simulink model "modelo_NL_DH_CL_pre_restauracao_2026-06-09"  (R2025b)
settings: Solver=ode4  StartTime=0.0  StopTime=60  FixedStep=SampleTime  RelTol=1e-3
undefined symbols (not defined in the file): att_alt, C_alt, C_phi, C_theta, C_vel, h_ref, h_step_final, h_step_init, h_step_t, K_heading, Kp, Kq, Kr, phi_step_final, phi_step_init, phi_step_t, psi_ref_final, psi_ref_init, psi_ref_t, theta_ref_clamp, theta_step_final, theta_step_init, theta_step_t, TrimInput, VT_ref, Xe
libraries: slpidlib x4
settings Model: SimulationMode=accelerator  Creator=anade  LastModifiedBy=kauemartinsdesouza
settings SolverCC: ZeroCrossAlgorithm=Adaptive
settings DebuggingCC: AlgebraicLoopMsg=none  IgnoredZcDiagnostic=none

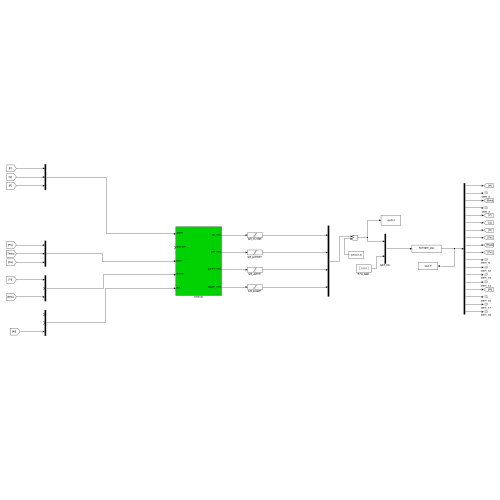
[thumbnail: Simulink's stored preview of the top-level diagram]
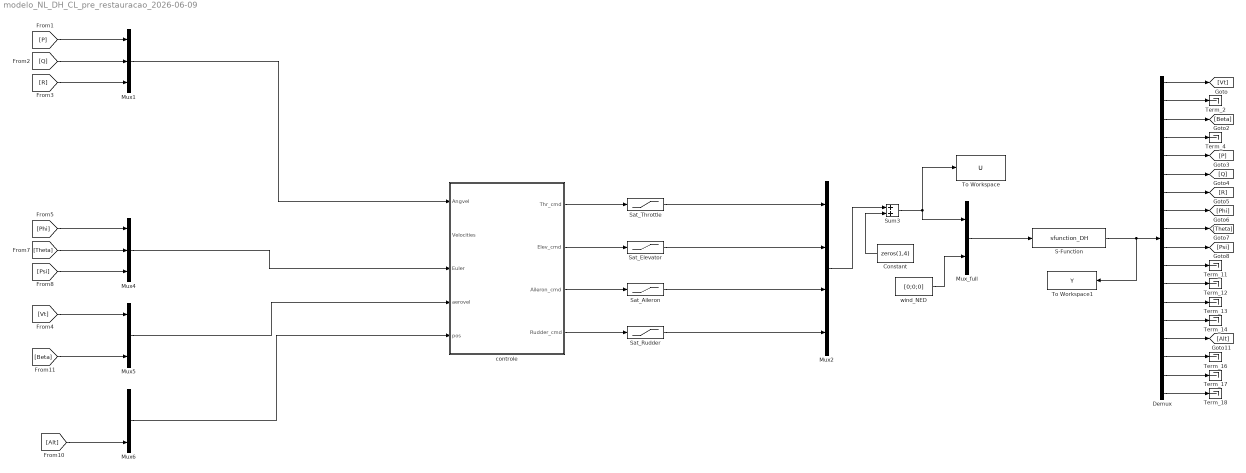
== system modelo_NL_DH_CL_pre_restauracao_2026-06-09 ==
  Constant : Constant  Value=zeros(1,4)
  Demux : Demux  Outputs=18
  Mux{1,4..6} (4 alike) : Mux  Inputs=3
  Mux2 : Mux
  Mux_full : Mux  Inputs=2
  S-Function : S-Function  FunctionName=sfunction_DH  Parameters=Xe  SFunctionDeploymentMode=off  EnableBusSupport=off
  Sat_Aileron : Saturate  UpperLimit=0.4363  LowerLimit=-0.4363
  Sat_Elevator : Saturate  UpperLimit=0.4363  LowerLimit=-0.4363
  Sat_Rudder : Saturate  UpperLimit=0.4363  LowerLimit=-0.4363
  Sat_Throttle : Saturate  UpperLimit=1  LowerLimit=0
  Sum3 : Sum
  Term_{2,4,11..14,16..18} (9 alike) : Terminator
  To Workspace : ToWorkspace  VariableName=U  SaveFormat=Structure With Time  SampleTime=-1
  To Workspace1 : ToWorkspace  VariableName=Y  SaveFormat=Structure With Time  SampleTime=-1
  controle : Subsystem
  wind_NED : Constant  Value=[0;0;0]
  wires:
  [Theta] -> Mux4/2
  Mux1/1 -> controle/1(Angvel)
  [Alt] -> Mux6/3
  [P] -> Mux1/1
  Mux4/1 -> controle/3(Euler)
  [R] -> Mux1/3
  [Phi] -> Mux4/1
  Mux6/1 -> controle/5(pos)
  [Q] -> Mux1/2
  Mux5/1 -> controle/4(aerovel)
  [Psi] -> Mux4/3
  [Beta] -> Mux5/3
  [Vt] -> Mux5/1
  controle/1(Thr_cmd) -> Sat_Throttle/1
  controle/2(Elev_cmd) -> Sat_Elevator/1
  controle/3(Aileron_cmd) -> Sat_Aileron/1
  controle/4(Rudder_cmd) -> Sat_Rudder/1
  Sat_Throttle/1 -> Mux2/1
  Sat_Elevator/1 -> Mux2/2
  Sat_Aileron/1 -> Mux2/3
  Sat_Rudder/1 -> Mux2/4
  Mux2/1 -> Sum3/1
  Constant/1 -> Sum3/2
  Sum3/1 -> Mux_full/1, To Workspace/1
  wind_NED/1 -> Mux_full/2
  Mux_full/1 -> S-Function/1
  S-Function/1 -> Demux/1, To Workspace1/1
  Demux/1 -> [Vt]
  Demux/2 -> Term_2/1
  Demux/3 -> [Beta]
  Demux/4 -> Term_4/1
  Demux/5 -> [P]
  Demux/6 -> [Q]
  Demux/7 -> [R]
  Demux/8 -> [Phi]
  Demux/9 -> [Theta]
  Demux/10 -> [Psi]
  Demux/11 -> Term_11/1
  Demux/12 -> Term_12/1
  Demux/13 -> Term_13/1
  Demux/14 -> Term_14/1
  Demux/15 -> [Alt]
  Demux/16 -> Term_16/1
  Demux/17 -> Term_17/1
  Demux/18 -> Term_18/1

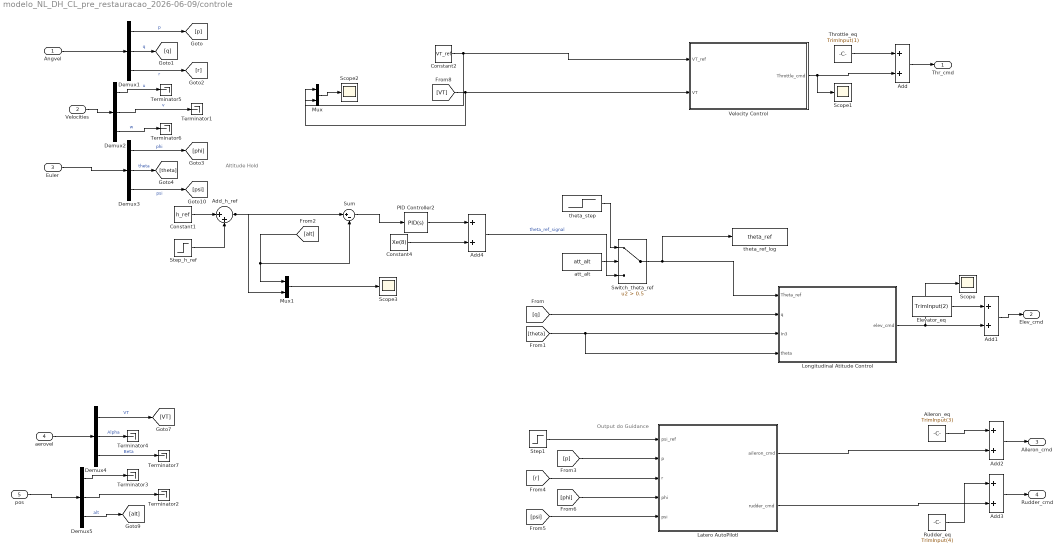
== system modelo_NL_DH_CL_pre_restauracao_2026-06-09/controle ==
  note: Altitude Hold
  note: Output do Guidance
  Angvel : Inport
  Velocities : Inport  Port=2
  Euler : Inport  Port=3
  aerovel : Inport  Port=4
  pos : Inport  Port=5
  Add{,1..4} (5 alike) : Sum
  Add_h_ref : Sum  Inputs=|++
  Aileron_eq : Constant  Value=TrimInput(3)
  Constant1 : Constant  Value=h_ref
  Constant2 : Constant  Value=VT_ref
  Constant4 : Constant  Value=Xe(8)
  Demux{1..5} (5 alike) : Demux  Outputs=3
  Elevator_eq : Constant  Value=TrimInput(2)
  Latero AutoPilotl : Subsystem
  Longitudinal Atitude Control : Subsystem
  Mux : Mux  Inputs=2
  Mux1 : Mux  Inputs=2
  PID Controller2 : slpidlib/PID Controller  Controller=PID  Form=Parallel  TimeDomain=Continuous-time  UseExternalTs=off  SampleTime=-1  IntegratorMethod=Forward Euler  FilterMethod=Forward Euler  ControllerParametersSource=internal  P=C_alt.Kp  I=C_alt.Ki  UseKiTs=off  D=C_alt.Kd  UseExternalDerivativeSource=off  N=C_alt.N  UseFilter=on  TunerSelectOption=Transfer Function Based (PID Tuner App)  InitialConditionSource=internal  InitialConditionForIntegrator=0  InitialConditionForFilter=0  DifferentiatorICPrevScaledInput=0  ExternalReset=none  TrackingMode=off  Kt=1  LimitOutput=on  SatLimitsSource=internal  UpperSaturationLimit=theta_ref_clamp(2)  LowerSaturationLimit=theta_ref_clamp(1)  LinearizeAsGain=on  AntiWindupMode=clamping  Kb=1  LimitIntegrator=off  UpperIntegratorSaturationLimit=inf  LowerIntegratorSaturationLimit=-inf  POutMin=[]  POutMax=[]  IOutMin=[]  IOutMax=[]  DOutMin=[]  DOutMax=[]  NOutMin=[]  NOutMax=[]  SumOutMin=[]  SumOutMax=[]  SaturationOutMin=[]  SaturationOutMax=[]  PParamMin=[]  PParamMax=[]  IParamMin=[]  IParamMax=[]  DParamMin=[]  DParamMax=[]  NParamMin=[]  NParamMax=[]  KbParamMin=[]  KbParamMax=[]  KtParamMin=[]  KtParamMax=[]  KbOutMin=[]  KbOutMax=[]  KtOutMin=[]  KtOutMax=[]  IntegratorOutMin=[]  IntegratorOutMax=[]  FilterOutMin=[]  FilterOutMax=[]  SumI1OutMin=[]  SumI1OutMax=[]  SumI2OutMin=[]  SumI2OutMax=[]  SumI3OutMin=[]  SumI3OutMax=[]  SumI4OutMin=[]  SumI4OutMax=[]  SumDOutMin=[]  SumDOutMax=[]  DifferentiatorOutMin=[]  DifferentiatorOutMax=[]  FilterDiffOutCoefMin=[]  FilterDiffOutCoefMax=[]  ReciprocalOutMin=[]  ReciprocalOutMax=[]  SumDenOutMin=[]  SumDenOutMax=[]  SumNumOutMin=[]  SumNumOutMax=[]  DivideOutMin=[]  DivideOutMax=[]  UdiffTsProdOutMin=[]  UdiffTsProdOutMax=[]  NTsProdOutMin=[]  NTsProdOutMax=[]  UintegralTsProdOutMin=[]  UintegralTsProdOutMax=[]  UngainTsProdOutMin=[]  UngainTsProdOutMax=[]  ClampingZeroOutDataTypeStr=Inherit: Inherit via back propagation  ClampingZeroOutMin=[]  ClampingZeroOutMax=[]  FilterDenConstantOutDataTypeStr=Inherit: Inherit via back propagation  FilterDenConstantOutMin=[]  FilterDenConstantOutMax=[]  PCopyOutDataTypeStr=Inherit: Inherit via back propagation  PCopyOutMin=[]  PCopyOutMax=[]  NCopyOutDataTypeStr=Inherit: Inherit via back propagation  NCopyOutMin=[]  NCopyOutMax=[]  IntegratorContinuousStateAttributes=''  IntegratorStateMustResolveToSignalObject=off  IntegratorRTWStateStorageClass=Auto  FilterContinuousStateAttributes=''  FilterStateMustResolveToSignalObject=off  FilterRTWStateStorageClass=Auto  ParallelPVariant=InternalParameters  IdealPVariant=Disabled  IVariant=InternalParameters  DVariant=InternalParameters  IntegratorVariant=Continuous  SatVariant=Enabled  AWVariant=ContClampingParallel  PCopyVariant=Disabled  TRVariant=Disabled  FdbkBlocksVariant=Forward  IdealPFdbkVariant=Disabled  SatFdbkVariant=Disabled  DerivativeFilterVariant=ContFilter  NVariant=InternalParameters  NCopyVariant=Disabled  FilterICVariant=InternalICsFilter  IntegratorICVariant=InternalICs  ExternalResetVariant=Disabled  TRSumVariant=Passthrough  SumFdbkVariant=Disabled  SumVariant=Sum_PID  TsampFilterVariant=InternalTs  TsampNgainVariant=Passthrough  TsampIntegralVariant=Disabled_SignalSpec  ExternalSaturationOutDataTypeStr=Inherit: Same as second input  DerivativeSourceVariant=ErrorSignal  PreIntVariant=InternalPreInt
  Rudder_eq : Constant  Value=TrimInput(4)
  Scope{,1..3} (4 alike) : Scope
      Scope settings: ActiveDisplayYMinimum=-1E-5  ActiveDisplayYMaximum=0.0001
      Scope1 settings: ActiveDisplayYMinimum=-746.9186  ActiveDisplayYMaximum=116.1605  DataLoggingVariableName=ScopeData2
      Scope2 settings: ActiveDisplayYMinimum=-70.825855594492936  ActiveDisplayYMaximum=79.160614638107518  DataLoggingVariableName=ScopeData4
      Scope3 settings: ActiveDisplayYMinimum=597.76222665286957  ActiveDisplayYMaximum=600.92459404043439  DataLoggingVariableName=ScopeData6
  Step1 : Step  Time=psi_ref_t  Before=psi_ref_init  After=psi_ref_final  SampleTime=0
  Step_h_ref : Step  Time=h_step_t  Before=h_step_init  After=h_step_final  SampleTime=0
  Sum : Sum  Inputs=|+-
  Switch_theta_ref : Switch  Criteria=u2 > Threshold  Threshold=0.5  SaturateOnIntegerOverflow=off  InputSameDT=off
  Terminator{1..7} (7 alike) : Terminator
  Throttle_eq : Constant  Value=TrimInput(1)
  Velocity Control : Subsystem
  att_alt : Constant  Value=att_alt
  theta_ref_log : ToWorkspace  VariableName=theta_ref  SaveFormat=Structure With Time  SampleTime=-1
  theta_step : Step  Time=theta_step_t  Before=theta_step_init  After=theta_step_final  SampleTime=0
  Thr_cmd : Outport
  Elev_cmd : Outport  Port=2
  Aileron_cmd : Outport  Port=3
  Rudder_cmd : Outport  Port=4
  wires:
  Angvel/1 -> Demux1/1
  Velocities/1 -> Demux2/1
  Demux1/1 -> [p]  "p"
  Demux1/2 -> [q]  "q"
  Demux1/3 -> [r]  "r"
  Euler/1 -> Demux3/1
  Demux3/3 -> [psi]  "psi"
  Demux3/1 -> [phi]  "phi"
  Demux3/2 -> [theta]  "theta"
  Demux2/3 -> Terminator6/1  "w"
  Demux2/1 -> Terminator5/1  "u"
  Demux2/2 -> Terminator1/1  "v"
  [theta] -> Longitudinal Atitude Control/3(In3), Longitudinal Atitude Control/4(theta)
  aerovel/1 -> Demux4/1
  Demux4/1 -> [VT]  "VT"
  Demux4/2 -> Terminator4/1  "Alpha"
  Demux4/3 -> Terminator7/1  "Beta"
  [q] -> Longitudinal Atitude Control/2(q)
  [VT] -> Mux/2, Velocity Control/2(VT)
  pos/1 -> Demux5/1
  Demux5/3 -> [alt]  "alt"
  Demux5/2 -> Terminator2/1
  Demux5/1 -> Terminator3/1
  [alt] -> Mux1/1, Sum/2
  [p] -> Latero AutoPilotl/2(p)
  [r] -> Latero AutoPilotl/3(r)
  [psi] -> Latero AutoPilotl/5(psi)
  [phi] -> Latero AutoPilotl/4(phi)
  Constant4/1 -> Add4/2
  Step1/1 -> Latero AutoPilotl/1(psi_ref)
  Mux/1 -> Scope2/1
  Add1/1 -> Elev_cmd/1
  Longitudinal Atitude Control/1(elev_cmd) -> Scope/1, Add1/2
  Add/1 -> Thr_cmd/1
  Velocity Control/1(Throttle_cmd) -> Scope1/1, Add/2
  Latero AutoPilotl/1(aileron_cmd) -> Add2/2
  Elevator_eq/1 -> Add1/1
  Rudder_eq/1 -> Add3/1
  Aileron_eq/1 -> Add2/1
  Latero AutoPilotl/2(rudder_cmd) -> Add3/2
  Add2/1 -> Aileron_cmd/1
  Add3/1 -> Rudder_cmd/1
  Throttle_eq/1 -> Add/1
  Mux1/1 -> Scope3/1
  Sum/1 -> PID Controller2/1
  PID Controller2/1 -> Add4/1
  Constant2/1 -> Mux/1, Velocity Control/1(VT_ref)
  theta_step/1 -> Switch_theta_ref/1
  att_alt/1 -> Switch_theta_ref/2
  Add4/1 -> Switch_theta_ref/3  "theta_ref_signal"
  Switch_theta_ref/1 -> Longitudinal Atitude Control/1(Theta_ref), theta_ref_log/1
  Add_h_ref/1 -> Sum/1, Mux1/2
  Constant1/1 -> Add_h_ref/1
  Step_h_ref/1 -> Add_h_ref/2

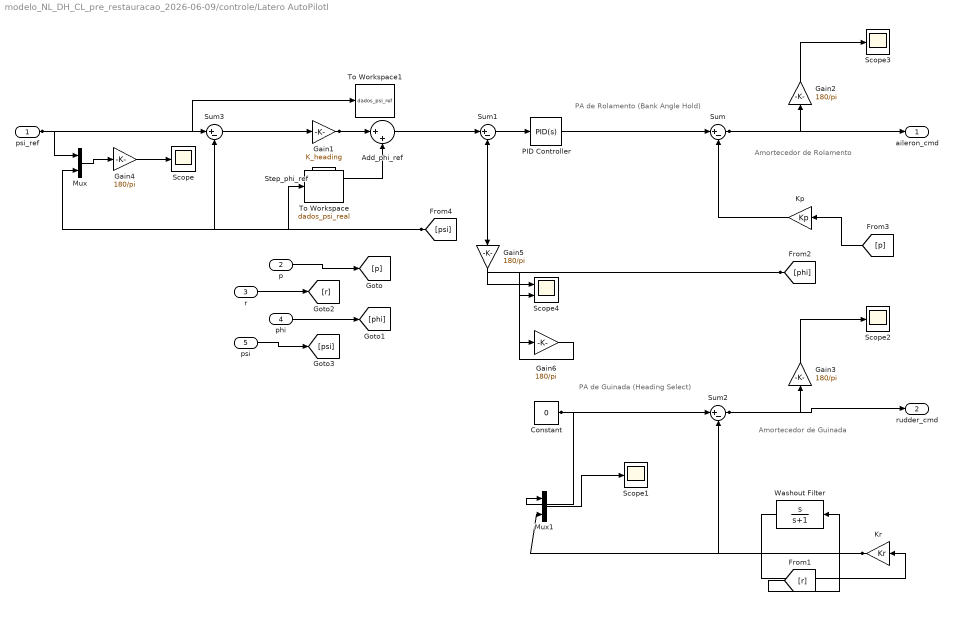
== system modelo_NL_DH_CL_pre_restauracao_2026-06-09/controle/Latero AutoPilotl ==
  note: PA de Rolamento (Bank Angle Hold)
  note: Amortecedor de Rolamento
  note: Amortecedor de Guinada
  note: PA de Guinada (Heading Select)
  psi_ref : Inport
  p : Inport  Port=2
  r : Inport  Port=3
  phi : Inport  Port=4
  psi : Inport  Port=5
  Add_phi_ref : Sum  Inputs=|++
  Constant : Constant  Value=0
  Gain1 : Gain  Gain=K_heading
  Gain{2..6} (5 alike) : Gain  Gain=180/pi
  Kp : Gain  Gain=Kp
  Kr : Gain  Gain=Kr
  Mux : Mux  Inputs=2
  Mux1 : Mux  Inputs=2
  PID Controller : slpidlib/PID Controller  Controller=PID  Form=Parallel  TimeDomain=Continuous-time  UseExternalTs=off  SampleTime=-1  IntegratorMethod=Forward Euler  FilterMethod=Forward Euler  ControllerParametersSource=internal  P=C_phi.Kp  I=C_phi.Ki  UseKiTs=off  D=C_phi.Kd  UseExternalDerivativeSource=off  N=C_phi.N  UseFilter=on  TunerSelectOption=Transfer Function Based (PID Tuner App)  InitialConditionSource=internal  InitialConditionForIntegrator=0  InitialConditionForFilter=0  DifferentiatorICPrevScaledInput=0  ExternalReset=none  TrackingMode=off  Kt=1  LimitOutput=on  SatLimitsSource=internal  UpperSaturationLimit=0.4363  LowerSaturationLimit=-0.4363  LinearizeAsGain=on  AntiWindupMode=clamping  Kb=1  LimitIntegrator=off  UpperIntegratorSaturationLimit=inf  LowerIntegratorSaturationLimit=-inf  POutMin=[]  POutMax=[]  IOutMin=[]  IOutMax=[]  DOutMin=[]  DOutMax=[]  NOutMin=[]  NOutMax=[]  SumOutMin=[]  SumOutMax=[]  SaturationOutMin=[]  SaturationOutMax=[]  PParamMin=[]  PParamMax=[]  IParamMin=[]  IParamMax=[]  DParamMin=[]  DParamMax=[]  NParamMin=[]  NParamMax=[]  KbParamMin=[]  KbParamMax=[]  KtParamMin=[]  KtParamMax=[]  KbOutMin=[]  KbOutMax=[]  KtOutMin=[]  KtOutMax=[]  IntegratorOutMin=[]  IntegratorOutMax=[]  FilterOutMin=[]  FilterOutMax=[]  SumI1OutMin=[]  SumI1OutMax=[]  SumI2OutMin=[]  SumI2OutMax=[]  SumI3OutMin=[]  SumI3OutMax=[]  SumI4OutMin=[]  SumI4OutMax=[]  SumDOutMin=[]  SumDOutMax=[]  DifferentiatorOutMin=[]  DifferentiatorOutMax=[]  FilterDiffOutCoefMin=[]  FilterDiffOutCoefMax=[]  ReciprocalOutMin=[]  ReciprocalOutMax=[]  SumDenOutMin=[]  SumDenOutMax=[]  SumNumOutMin=[]  SumNumOutMax=[]  DivideOutMin=[]  DivideOutMax=[]  UdiffTsProdOutMin=[]  UdiffTsProdOutMax=[]  NTsProdOutMin=[]  NTsProdOutMax=[]  UintegralTsProdOutMin=[]  UintegralTsProdOutMax=[]  UngainTsProdOutMin=[]  UngainTsProdOutMax=[]  ClampingZeroOutDataTypeStr=Inherit: Inherit via back propagation  ClampingZeroOutMin=[]  ClampingZeroOutMax=[]  FilterDenConstantOutDataTypeStr=Inherit: Inherit via back propagation  FilterDenConstantOutMin=[]  FilterDenConstantOutMax=[]  PCopyOutDataTypeStr=Inherit: Inherit via back propagation  PCopyOutMin=[]  PCopyOutMax=[]  NCopyOutDataTypeStr=Inherit: Inherit via back propagation  NCopyOutMin=[]  NCopyOutMax=[]  IntegratorContinuousStateAttributes=''  IntegratorStateMustResolveToSignalObject=off  IntegratorRTWStateStorageClass=Auto  FilterContinuousStateAttributes=''  FilterStateMustResolveToSignalObject=off  FilterRTWStateStorageClass=Auto  ParallelPVariant=InternalParameters  IdealPVariant=Disabled  IVariant=InternalParameters  DVariant=InternalParameters  IntegratorVariant=Continuous  SatVariant=Enabled  AWVariant=ContClampingParallel  PCopyVariant=Disabled  TRVariant=Disabled  FdbkBlocksVariant=Forward  IdealPFdbkVariant=Disabled  SatFdbkVariant=Disabled  DerivativeFilterVariant=ContFilter  NVariant=InternalParameters  NCopyVariant=Disabled  FilterICVariant=InternalICsFilter  IntegratorICVariant=InternalICs  ExternalResetVariant=Disabled  TRSumVariant=Passthrough  SumFdbkVariant=Disabled  SumVariant=Sum_PID  TsampFilterVariant=InternalTs  TsampNgainVariant=Passthrough  TsampIntegralVariant=Disabled_SignalSpec  ExternalSaturationOutDataTypeStr=Inherit: Same as second input  DerivativeSourceVariant=ErrorSignal  PreIntVariant=InternalPreInt
  Scope{,1..3} (4 alike) : Scope
      Scope settings: ActiveDisplayYMinimum=-9.73683  ActiveDisplayYMaximum=51.08187  DataLoggingVariableName=ScopeData5
      Scope1 settings: ActiveDisplayYMinimum=-0.53028169211297194  ActiveDisplayYMaximum=0.24100187800441716
      Scope2 settings: ActiveDisplayYMinimum=-4.64142  ActiveDisplayYMaximum=2.08449
      Scope3 settings: ActiveDisplayYMinimum=-384.74036  ActiveDisplayYMaximum=1108.75141  DataLoggingVariableName=ScopeData2
  Scope4 : Scope  NumInputPorts=2
      settings: ActiveDisplayYMinimum=-4.8655  ActiveDisplayYMaximum=43.78946  DataLoggingVariableName=ScopeData3
  Step_phi_ref : Step  Time=phi_step_t  Before=phi_step_init  After=phi_step_final  SampleTime=0
  Sum{,1..3} (4 alike) : Sum  Inputs=|+-
  To Workspace : ToWorkspace  VariableName=dados_psi_real  SaveFormat=Timeseries  SampleTime=-1
      settings: Save2DSignal=2-D array (concatenate along first dimension)
  To Workspace1 : ToWorkspace  VariableName=dados_psi_ref  SaveFormat=Timeseries  SampleTime=-1
      settings: Save2DSignal=2-D array (concatenate along first dimension)
  Washout Filter : TransferFcn  Numerator=[1 0]  Denominator=[1 1]
  aileron_cmd : Outport
  rudder_cmd : Outport  Port=2
  wires:
  Sum1/1 -> PID Controller/1
  Sum/1 -> Gain2/1, aileron_cmd/1
  [p] -> Kp/1
  [phi] -> Sum1/2, Gain6/1
  Kp/1 -> Sum/2
  PID Controller/1 -> Sum/1
  p/1 -> [p]
  [r] -> Washout Filter/1
  Kr/1 -> Mux1/2, Sum2/2
  r/1 -> [r]
  Washout Filter/1 -> Kr/1
  phi/1 -> [phi]
  psi/1 -> [psi]
  Sum3/1 -> Gain1/1
  [psi] -> To Workspace/1, Sum3/2, Mux/2
  psi_ref/1 -> Mux/1, To Workspace1/1, Sum3/1
  Sum2/1 -> Gain3/1, rudder_cmd/1
  Constant/1 -> Mux1/1, Sum2/1
  Gain1/1 -> Gain5/1, Add_phi_ref/1
  Mux/1 -> Gain4/1
  Mux1/1 -> Scope1/1
  Gain2/1 -> Scope3/1
  Gain3/1 -> Scope2/1
  Gain4/1 -> Scope/1
  Gain5/1 -> Scope4/1
  Gain6/1 -> Scope4/2
  Step_phi_ref/1 -> Add_phi_ref/2
  Add_phi_ref/1 -> Sum1/1

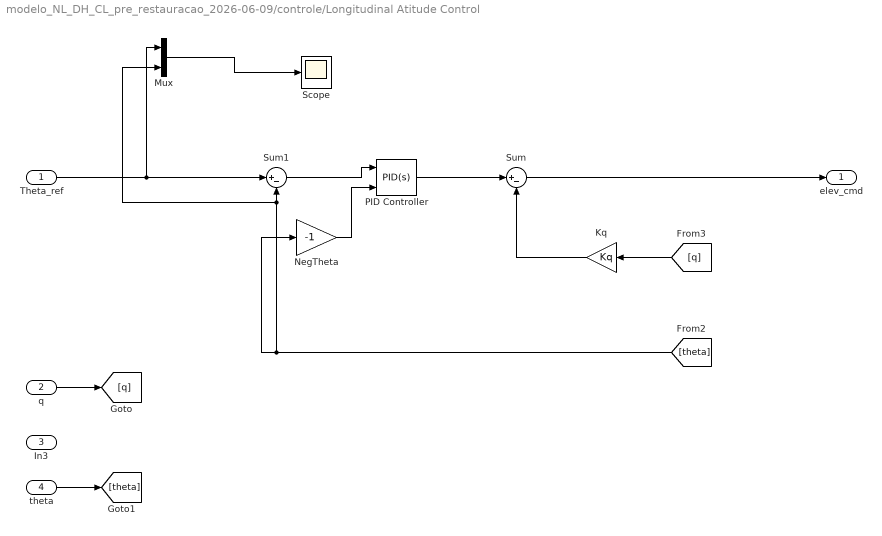
== system modelo_NL_DH_CL_pre_restauracao_2026-06-09/controle/Longitudinal Atitude Control ==
  Theta_ref : Inport
  q : Inport  Port=2
  In3 : Inport  Port=3
  theta : Inport  Port=4
  Kq : Gain  Gain=Kq
  Mux : Mux  Inputs=2
  NegTheta : Gain  Gain=-1
  PID Controller : slpidlib/PID Controller  Controller=PID  Form=Parallel  TimeDomain=Continuous-time  UseExternalTs=off  SampleTime=-1  IntegratorMethod=Forward Euler  FilterMethod=Forward Euler  ControllerParametersSource=internal  P=C_theta.Kp  I=C_theta.Ki  UseKiTs=off  D=C_theta.Kd  UseExternalDerivativeSource=on  N=C_theta.N  UseFilter=on  TunerSelectOption=Transfer Function Based (PID Tuner App)  InitialConditionSource=internal  InitialConditionForIntegrator=0  InitialConditionForFilter=0  DifferentiatorICPrevScaledInput=0  ExternalReset=none  TrackingMode=off  Kt=1  LimitOutput=on  SatLimitsSource=internal  UpperSaturationLimit=0.4363  LowerSaturationLimit=-0.4363  LinearizeAsGain=on  AntiWindupMode=clamping  Kb=1  LimitIntegrator=off  UpperIntegratorSaturationLimit=inf  LowerIntegratorSaturationLimit=-inf  POutMin=[]  POutMax=[]  IOutMin=[]  IOutMax=[]  DOutMin=[]  DOutMax=[]  NOutMin=[]  NOutMax=[]  SumOutMin=[]  SumOutMax=[]  SaturationOutMin=[]  SaturationOutMax=[]  PParamMin=[]  PParamMax=[]  IParamMin=[]  IParamMax=[]  DParamMin=[]  DParamMax=[]  NParamMin=[]  NParamMax=[]  KbParamMin=[]  KbParamMax=[]  KtParamMin=[]  KtParamMax=[]  KbOutMin=[]  KbOutMax=[]  KtOutMin=[]  KtOutMax=[]  IntegratorOutMin=[]  IntegratorOutMax=[]  FilterOutMin=[]  FilterOutMax=[]  SumI1OutMin=[]  SumI1OutMax=[]  SumI2OutMin=[]  SumI2OutMax=[]  SumI3OutMin=[]  SumI3OutMax=[]  SumI4OutMin=[]  SumI4OutMax=[]  SumDOutMin=[]  SumDOutMax=[]  DifferentiatorOutMin=[]  DifferentiatorOutMax=[]  FilterDiffOutCoefMin=[]  FilterDiffOutCoefMax=[]  ReciprocalOutMin=[]  ReciprocalOutMax=[]  SumDenOutMin=[]  SumDenOutMax=[]  SumNumOutMin=[]  SumNumOutMax=[]  DivideOutMin=[]  DivideOutMax=[]  UdiffTsProdOutMin=[]  UdiffTsProdOutMax=[]  NTsProdOutMin=[]  NTsProdOutMax=[]  UintegralTsProdOutMin=[]  UintegralTsProdOutMax=[]  UngainTsProdOutMin=[]  UngainTsProdOutMax=[]  ClampingZeroOutDataTypeStr=Inherit: Inherit via back propagation  ClampingZeroOutMin=[]  ClampingZeroOutMax=[]  FilterDenConstantOutDataTypeStr=Inherit: Inherit via back propagation  FilterDenConstantOutMin=[]  FilterDenConstantOutMax=[]  PCopyOutDataTypeStr=Inherit: Inherit via back propagation  PCopyOutMin=[]  PCopyOutMax=[]  NCopyOutDataTypeStr=Inherit: Inherit via back propagation  NCopyOutMin=[]  NCopyOutMax=[]  IntegratorContinuousStateAttributes=''  IntegratorStateMustResolveToSignalObject=off  IntegratorRTWStateStorageClass=Auto  FilterContinuousStateAttributes=''  FilterStateMustResolveToSignalObject=off  FilterRTWStateStorageClass=Auto  ParallelPVariant=InternalParameters  IdealPVariant=Disabled  IVariant=InternalParameters  DVariant=InternalParameters  IntegratorVariant=Continuous  SatVariant=Enabled  AWVariant=ContClampingParallel  PCopyVariant=Disabled  TRVariant=Disabled  FdbkBlocksVariant=Forward  IdealPFdbkVariant=Disabled  SatFdbkVariant=Disabled  DerivativeFilterVariant=ContFilterOnly  NVariant=InternalParameters  NCopyVariant=Disabled  FilterICVariant=InternalICsFilter  IntegratorICVariant=InternalICs  ExternalResetVariant=Disabled  TRSumVariant=Passthrough  SumFdbkVariant=Disabled  SumVariant=Sum_PID  TsampFilterVariant=InternalTs  TsampNgainVariant=Passthrough  TsampIntegralVariant=Disabled_SignalSpec  ExternalSaturationOutDataTypeStr=Inherit: Same as second input  DerivativeSourceVariant=ExternalYdot  PreIntVariant=InternalPreInt
  Scope : Scope
      settings: ActiveDisplayYMinimum=-0.015348297793364607  ActiveDisplayYMaximum=0.13813468014028149  DataLoggingVariableName=ScopeData3
  Sum : Sum  Inputs=|+-
  Sum1 : Sum  Inputs=|+-
  elev_cmd : Outport
  wires:
  Sum1/1 -> PID Controller/1
  Sum/1 -> elev_cmd/1
  [q] -> Kq/1
  [theta] -> Mux/2, Sum1/2, NegTheta/1
  Kq/1 -> Sum/2
  PID Controller/1 -> Sum/1
  theta/1 -> [theta]
  q/1 -> [q]
  Theta_ref/1 -> Mux/1, Sum1/1
  Mux/1 -> Scope/1
  NegTheta/1 -> PID Controller/2

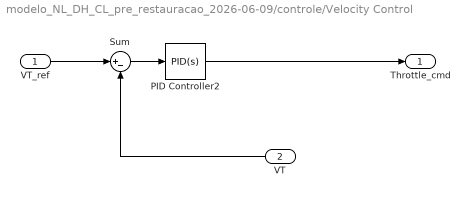
== system modelo_NL_DH_CL_pre_restauracao_2026-06-09/controle/Velocity Control ==
  VT_ref : Inport
  VT : Inport  Port=2
  PID Controller2 : slpidlib/PID Controller  Controller=PID  Form=Parallel  TimeDomain=Continuous-time  UseExternalTs=off  SampleTime=-1  IntegratorMethod=Forward Euler  FilterMethod=Forward Euler  ControllerParametersSource=internal  P=C_vel.Kp  I=C_vel.Ki  UseKiTs=off  D=C_vel.Kd  UseExternalDerivativeSource=off  N=C_vel.N  UseFilter=on  TunerSelectOption=Transfer Function Based (PID Tuner App)  InitialConditionSource=internal  InitialConditionForIntegrator=0  InitialConditionForFilter=0  DifferentiatorICPrevScaledInput=0  ExternalReset=none  TrackingMode=off  Kt=1  LimitOutput=on  SatLimitsSource=internal  UpperSaturationLimit=0.51  LowerSaturationLimit=-0.49  LinearizeAsGain=on  AntiWindupMode=clamping  Kb=1  LimitIntegrator=off  UpperIntegratorSaturationLimit=inf  LowerIntegratorSaturationLimit=-inf  POutMin=[]  POutMax=[]  IOutMin=[]  IOutMax=[]  DOutMin=[]  DOutMax=[]  NOutMin=[]  NOutMax=[]  SumOutMin=[]  SumOutMax=[]  SaturationOutMin=[]  SaturationOutMax=[]  PParamMin=[]  PParamMax=[]  IParamMin=[]  IParamMax=[]  DParamMin=[]  DParamMax=[]  NParamMin=[]  NParamMax=[]  KbParamMin=[]  KbParamMax=[]  KtParamMin=[]  KtParamMax=[]  KbOutMin=[]  KbOutMax=[]  KtOutMin=[]  KtOutMax=[]  IntegratorOutMin=[]  IntegratorOutMax=[]  FilterOutMin=[]  FilterOutMax=[]  SumI1OutMin=[]  SumI1OutMax=[]  SumI2OutMin=[]  SumI2OutMax=[]  SumI3OutMin=[]  SumI3OutMax=[]  SumI4OutMin=[]  SumI4OutMax=[]  SumDOutMin=[]  SumDOutMax=[]  DifferentiatorOutMin=[]  DifferentiatorOutMax=[]  FilterDiffOutCoefMin=[]  FilterDiffOutCoefMax=[]  ReciprocalOutMin=[]  ReciprocalOutMax=[]  SumDenOutMin=[]  SumDenOutMax=[]  SumNumOutMin=[]  SumNumOutMax=[]  DivideOutMin=[]  DivideOutMax=[]  UdiffTsProdOutMin=[]  UdiffTsProdOutMax=[]  NTsProdOutMin=[]  NTsProdOutMax=[]  UintegralTsProdOutMin=[]  UintegralTsProdOutMax=[]  UngainTsProdOutMin=[]  UngainTsProdOutMax=[]  ClampingZeroOutDataTypeStr=Inherit: Inherit via back propagation  ClampingZeroOutMin=[]  ClampingZeroOutMax=[]  FilterDenConstantOutDataTypeStr=Inherit: Inherit via back propagation  FilterDenConstantOutMin=[]  FilterDenConstantOutMax=[]  PCopyOutDataTypeStr=Inherit: Inherit via back propagation  PCopyOutMin=[]  PCopyOutMax=[]  NCopyOutDataTypeStr=Inherit: Inherit via back propagation  NCopyOutMin=[]  NCopyOutMax=[]  IntegratorContinuousStateAttributes=''  IntegratorStateMustResolveToSignalObject=off  IntegratorRTWStateStorageClass=Auto  FilterContinuousStateAttributes=''  FilterStateMustResolveToSignalObject=off  FilterRTWStateStorageClass=Auto  ParallelPVariant=InternalParameters  IdealPVariant=Disabled  IVariant=InternalParameters  DVariant=InternalParameters  IntegratorVariant=Continuous  SatVariant=Enabled  AWVariant=ContClampingParallel  PCopyVariant=Disabled  TRVariant=Disabled  FdbkBlocksVariant=Forward  IdealPFdbkVariant=Disabled  SatFdbkVariant=Disabled  DerivativeFilterVariant=ContFilter  NVariant=InternalParameters  NCopyVariant=Disabled  FilterICVariant=InternalICsFilter  IntegratorICVariant=InternalICs  ExternalResetVariant=Disabled  TRSumVariant=Passthrough  SumFdbkVariant=Disabled  SumVariant=Sum_PID  TsampFilterVariant=InternalTs  TsampNgainVariant=Passthrough  TsampIntegralVariant=Disabled_SignalSpec  ExternalSaturationOutDataTypeStr=Inherit: Same as second input  DerivativeSourceVariant=ErrorSignal  PreIntVariant=InternalPreInt
  Sum : Sum  Inputs=|+-
  Throttle_cmd : Outport
  wires:
  VT/1 -> Sum/2
  PID Controller2/1 -> Throttle_cmd/1
  VT_ref/1 -> Sum/1
  Sum/1 -> PID Controller2/1
